simulink model "PubIfDecisionLM_MDL"  (R2020b)
settings: configuration reference "DspaceConfig" (kept outside this file)
PostLoadFcn:
  | if any(exist('dsrtsu_mdlpostloadfcn', 'file') ~= 0), dsrtsu_mdlpostloadfcn('Execute', bdroot); end
InitFcn:
  | , if any(exist('dsmpb_private', 'file') ~= 0), dsmpb_private('dsmpb_mdlclblib', 'Init', bdroot); end,
undefined symbols (not defined in the file or in its folder): OFM_OBJ_FUSIONTYPE_E, OFM_OBJ_MOVINGSTATE_E, OFM_OBJ_ORIENTATION_E, OFM_OBJ_TYPE_E, P_LM_Cyc, P_LM_EMLHistKapRcdBufSize, P_LM_EMLHistTrajBaseDis, P_LM_EMLHistTrajPNum, P_LM_EMLKapCorrMaxThre, P_LM_EMLMinKapThre, P_LM_EMLPathDisDiffThre, P_LM_EMLQuaFiltPar, P_LM_EMLTurnActKapThre, P_LM_EMLValidQuaThre, P_LM_FntPath1Disgap, P_LM_FntPath1MinDis, P_LM_FntPath1Timegap, P_LM_FntPath2Disgap, P_LM_FntPath2MinDis, P_LM_FntPath2Timegap, P_LM_FntPath3Disgap, P_LM_FntPath3MinDis, P_LM_FntPath3Timegap, P_LM_FusBLParFiltP, P_LM_FusEVDifC2Thre, P_LM_FusEVOPath1AllVSLDisThre, P_LM_FusEVOPath1AllVSLLostNumThre, P_LM_FusEVOPath1AllVSLQuaThre, P_LM_FusEVOPath1OTLFacNLC, P_LM_FusOTLQuaThre, P_LM_FusOTLSW, P_LM_FusParC0Index, P_LM_FusParC1Index, P_LM_FusParC2Index, P_LM_FusParC3Index, P_LM_FusVSLQuaThre, P_LM_FusVSLSW, P_LM_FusVSLValidSteerWheerAngThre, P_LM_FusVSLValidVxvThre, P_LM_LaneWidth, P_LM_OTLBufTPInfoEvaFactor, P_LM_OTLObjNum, P_LM_OTLObjSelectAgeThre, P_LM_OTLObjSelectDxAssessVx, P_LM_OTLObjSelectDxThre, P_LM_OTLObjSelectVxThre, P_LM_OTLObjSelectVyAssessDx, P_LM_OTLObjSelectVyThre, P_LM_OTLTrajPntBaseDis, P_LM_OTLTrajStdThre, P_LM_VSLAvailLineNum, P_LM_VSLBLSDiffThre, P_LM_VSLBLSDisRatio, P_LM_VSLFusBLParFiltP_C1, P_LM_VSLFusBLParFiltP_C2, P_LM_VSLFusBLParFiltP_C3, P_LM_VSLFusBLParFiltP_Quality, P_LM_VSLHistTrajBaseDis, P_LM_VSLHistTrajPNum, P_LM_VSLLCC0diff ... (+18)
libraries: simulink x145, LM_LIB x43
(part 15 of 24)

== system PubIfDecisionLM_MDL/Subsystem2/LM_Fusion1/LM_Fus_BLConnectivityCheck/LM_Fus_BLFntPahtConnectivityCheck/LM_Fus_BLFntPahtConnectivityCheck/LM_Fus_BLFntPath2Info/LM_Fus_BLFntPath2C0Adju ==
  LM_FusBLFntPath1C0 : Inport
  LM_FusBLFntPath1C1 : Inport  Port=2
  LM_FusBLFntPath1C2 : Inport  Port=3
  LM_FusBLFntPath1C3 : Inport  Port=4
  LM_FntPath1Dis : Inport  Port=5
  LM_FusBLFntPath2C0BefAduj : Inport  Port=6
  LM_FusBLFntPath2C1 : Inport  Port=7
  LM_FusBLFntPath2C2 : Inport  Port=8
  LM_FusBLFntPath2C3 : Inport  Port=9
  LM_Fus_BLFntPaht1EndPosCalc : Subsystem
  LM_Fus_BLFntPath2C0Adju : Subsystem
  LM_Fus_BLFntPath2StartPosCalc : Subsystem
  LM_FusBLFntPath2C0Aduj : Outport
  wires:
  LM_FusBLFntPath1C0/1 -> LM_Fus_BLFntPaht1EndPosCalc/1(LM_FusBLFntPath1C0)
  LM_FusBLFntPath1C1/1 -> LM_Fus_BLFntPaht1EndPosCalc/2(LM_FusBLFntPath1C1)
  LM_FusBLFntPath1C2/1 -> LM_Fus_BLFntPaht1EndPosCalc/3(LM_FusBLFntPath1C2)
  LM_FusBLFntPath1C3/1 -> LM_Fus_BLFntPaht1EndPosCalc/4(LM_FusBLFntPath1C3)
  LM_FntPath1Dis/1 -> LM_Fus_BLFntPath2StartPosCalc/1(LM_FntPath1Dis), LM_Fus_BLFntPaht1EndPosCalc/5(LM_FntPath1Dis)
  LM_FusBLFntPath2C1/1 -> LM_Fus_BLFntPath2StartPosCalc/2(LM_FusBLFntPath2C1)
  LM_FusBLFntPath2C2/1 -> LM_Fus_BLFntPath2StartPosCalc/3(LM_FusBLFntPath2C2)
  LM_FusBLFntPath2C3/1 -> LM_Fus_BLFntPath2StartPosCalc/4(LM_FusBLFntPath2C3)
  LM_FusBLFntPath2C0BefAduj/1 -> LM_Fus_BLFntPath2C0Adju/3(LM_FusBLFntPath2C0BefAduj), LM_Fus_BLFntPath2StartPosCalc/5(LM_FusBLFntPath2C0BefAduj)
  LM_Fus_BLFntPaht1EndPosCalc/1(LM_FusBLFntPaht1EndPosdy) -> LM_Fus_BLFntPath2C0Adju/1(LM_FusBLFntPaht1EndPosdy)
  LM_Fus_BLFntPath2StartPosCalc/1(LM_FusBLFntPaht2StartPosdy) -> LM_Fus_BLFntPath2C0Adju/2(LM_FusBLFntPaht2StartPosdy)
  LM_Fus_BLFntPath2C0Adju/1(LM_FusBLFntPath2C0Aduj) -> LM_FusBLFntPath2C0Aduj/1

== system PubIfDecisionLM_MDL/Subsystem2/LM_Fusion1/LM_Fus_BLConnectivityCheck/LM_Fus_BLFntPahtConnectivityCheck/LM_Fus_BLFntPahtConnectivityCheck/LM_Fus_BLFntPath2Info/LM_Fus_BLFntPath2Info ==
  LM_FusBLFntPath2C0Aduj : Inport
  LM_FusBLFntPath2C1 : Inport  Port=2
  LM_FusBLFntPath2C2 : Inport  Port=3
  LM_FusBLFntPath2C3 : Inport  Port=4
  LM_FusBLFntPath2Quality : Inport  Port=5
  Signal Conversion{,1..4} (5 alike) : SignalConversion  OverrideOpt=off
  LM_FusBLFntPath2C0Adju : Outport
  LM_FusBLFntPath2C1Adju : Outport  Port=2
  LM_FusBLFntPath2C2Adju : Outport  Port=3
  LM_FusBLFntPath2C3Adju : Outport  Port=4
  LM_FusBLFntPath2QualityAdju : Outport  Port=5
  wires:
  LM_FusBLFntPath2Quality/1 -> Signal Conversion4/1
  LM_FusBLFntPath2C2/1 -> Signal Conversion2/1
  LM_FusBLFntPath2C1/1 -> Signal Conversion1/1
  LM_FusBLFntPath2C0Aduj/1 -> Signal Conversion/1
  LM_FusBLFntPath2C3/1 -> Signal Conversion3/1
  Signal Conversion/1 -> LM_FusBLFntPath2C0Adju/1  "LM_FusBLFntPath2C0Adju"
  Signal Conversion2/1 -> LM_FusBLFntPath2C2Adju/1  "LM_FusBLFntPath2C2Adju"
  Signal Conversion4/1 -> LM_FusBLFntPath2QualityAdju/1  "LM_FusBLFntPath2QualityAdju"
  Signal Conversion3/1 -> LM_FusBLFntPath2C3Adju/1  "LM_FusBLFntPath2C3Adju"
  Signal Conversion1/1 -> LM_FusBLFntPath2C1Adju/1  "LM_FusBLFntPath2C1Adju"

== system PubIfDecisionLM_MDL/Subsystem2/LM_Fusion1/LM_Fus_BLConnectivityCheck/LM_Fus_BLFntPahtConnectivityCheck/LM_Fus_BLFntPahtConnectivityCheck/LM_Fus_BLFntPath3Info/LM_Fus_BLFntPath2C0Adju ==
  LM_FusBLFntPath2C0 : Inport
  LM_FusBLFntPath2C1 : Inport  Port=2
  LM_FusBLFntPath2C2 : Inport  Port=3
  LM_FusBLFntPath2C3 : Inport  Port=4
  LM_FntPath2Dis : Inport  Port=5
  LM_FusBLFntPath3C0BefAduj : Inport  Port=6
  LM_FusBLFntPath3C1 : Inport  Port=7
  LM_FusBLFntPath3C2 : Inport  Port=8
  LM_FusBLFntPath3C3 : Inport  Port=9
  LM_Fus_BLFntPaht2EndPosCalc : Subsystem
  LM_Fus_BLFntPath3C0Adju : Subsystem
  LM_Fus_BLFntPath3StartPosCalc : Subsystem
  LM_FusBLFntPath3C0Aduj : Outport
  wires:
  LM_FusBLFntPath2C0/1 -> LM_Fus_BLFntPaht2EndPosCalc/1(LM_FusBLFntPath2C0)
  LM_FusBLFntPath2C1/1 -> LM_Fus_BLFntPaht2EndPosCalc/2(LM_FusBLFntPath2C1)
  LM_FusBLFntPath2C2/1 -> LM_Fus_BLFntPaht2EndPosCalc/3(LM_FusBLFntPath2C2)
  LM_FusBLFntPath2C3/1 -> LM_Fus_BLFntPaht2EndPosCalc/4(LM_FusBLFntPath2C3)
  LM_FntPath2Dis/1 -> LM_Fus_BLFntPath3StartPosCalc/1(LM_FntPath2Dis), LM_Fus_BLFntPaht2EndPosCalc/5(LM_FntPath2Dis)
  LM_FusBLFntPath3C1/1 -> LM_Fus_BLFntPath3StartPosCalc/2(LM_FusBLFntPath3C1)
  LM_FusBLFntPath3C2/1 -> LM_Fus_BLFntPath3StartPosCalc/3(LM_FusBLFntPath3C2)
  LM_FusBLFntPath3C3/1 -> LM_Fus_BLFntPath3StartPosCalc/4(LM_FusBLFntPath3C3)
  LM_FusBLFntPath3C0BefAduj/1 -> LM_Fus_BLFntPath3C0Adju/3(LM_FusBLFntPath3C0BefAduj), LM_Fus_BLFntPath3StartPosCalc/5(LM_FusBLFntPath3C0BefAduj)
  LM_Fus_BLFntPaht2EndPosCalc/1(LM_FusBLFntPaht2EndPosdy) -> LM_Fus_BLFntPath3C0Adju/1(LM_FusBLFntPaht2EndPosdy)
  LM_Fus_BLFntPath3StartPosCalc/1(LM_FusBLFntPaht3StartPosdy) -> LM_Fus_BLFntPath3C0Adju/2(LM_FusBLFntPaht3StartPosdy)
  LM_Fus_BLFntPath3C0Adju/1(LM_FusBLFntPath3C0Aduj) -> LM_FusBLFntPath3C0Aduj/1

== system PubIfDecisionLM_MDL/Subsystem2/LM_Fusion1/LM_Fus_BLConnectivityCheck/LM_Fus_BLFntPahtConnectivityCheck/LM_Fus_BLFntPahtConnectivityCheck/LM_Fus_BLFntPath3Info/LM_Fus_BLFntPath2Info ==
  LM_FusBLFntPath3C0Aduj : Inport
  LM_FusBLFntPath3C1 : Inport  Port=2
  LM_FusBLFntPath3C2 : Inport  Port=3
  LM_FusBLFntPath3C3 : Inport  Port=4
  LM_FusBLFntPath3Quality : Inport  Port=5
  Signal Conversion{,1..4} (5 alike) : SignalConversion  OverrideOpt=off
  LM_FusBLFntPath3C0Adju : Outport
  LM_FusBLFntPath3C1Adju : Outport  Port=2
  LM_FusBLFntPath3C2Adju : Outport  Port=3
  LM_FusBLFntPath3C3Adju : Outport  Port=4
  LM_FusBLFntPath3QualityAdju : Outport  Port=5
  wires:
  Signal Conversion4/1 -> LM_FusBLFntPath3QualityAdju/1  "LM_FusBLFntPath3QualityAdju"
  Signal Conversion2/1 -> LM_FusBLFntPath3C2Adju/1  "LM_FusBLFntPath3C2Adju"
  Signal Conversion/1 -> LM_FusBLFntPath3C0Adju/1  "LM_FusBLFntPath3C0Adju"
  Signal Conversion3/1 -> LM_FusBLFntPath3C3Adju/1  "LM_FusBLFntPath3C3Adju"
  Signal Conversion1/1 -> LM_FusBLFntPath3C1Adju/1  "LM_FusBLFntPath3C1Adju"
  LM_FusBLFntPath3C0Aduj/1 -> Signal Conversion/1
  LM_FusBLFntPath3C1/1 -> Signal Conversion1/1
  LM_FusBLFntPath3C2/1 -> Signal Conversion2/1
  LM_FusBLFntPath3C3/1 -> Signal Conversion3/1
  LM_FusBLFntPath3Quality/1 -> Signal Conversion4/1

== system PubIfDecisionLM_MDL/Subsystem2/LM_Fusion1/LM_Fus_BLConnectivityCheck/LM_Fus_BLRearPahtConnectivityCheck/LM_Fus_BLRearPahtConnectivityCheck/LM_Fus_BLFntPath2Info/LM_Fus_BLFntPath2C0Adju ==
  LM_FusBLFntPath1C0 : Inport
  LM_FusBLFntPath1C1 : Inport  Port=2
  LM_FusBLFntPath1C2 : Inport  Port=3
  LM_FusBLFntPath1C3 : Inport  Port=4
  LM_FntPath1Dis : Inport  Port=5
  LM_FusBLFntPath2C0BefAduj : Inport  Port=6
  LM_FusBLFntPath2C1 : Inport  Port=7
  LM_FusBLFntPath2C2 : Inport  Port=8
  LM_FusBLFntPath2C3 : Inport  Port=9
  LM_Fus_BLFntPaht1EndPosCalc : Subsystem
  LM_Fus_BLFntPath2C0Adju : Subsystem
  LM_Fus_BLFntPath2StartPosCalc : Subsystem
  LM_FusBLFntPath2C0Aduj : Outport
  wires:
  LM_FusBLFntPath1C0/1 -> LM_Fus_BLFntPaht1EndPosCalc/1(LM_FusBLFntPath1C0)
  LM_FusBLFntPath1C1/1 -> LM_Fus_BLFntPaht1EndPosCalc/2(LM_FusBLFntPath1C1)
  LM_FusBLFntPath1C2/1 -> LM_Fus_BLFntPaht1EndPosCalc/3(LM_FusBLFntPath1C2)
  LM_FusBLFntPath1C3/1 -> LM_Fus_BLFntPaht1EndPosCalc/4(LM_FusBLFntPath1C3)
  LM_FntPath1Dis/1 -> LM_Fus_BLFntPath2StartPosCalc/1(LM_FntPath1Dis), LM_Fus_BLFntPaht1EndPosCalc/5(LM_FntPath1Dis)
  LM_FusBLFntPath2C1/1 -> LM_Fus_BLFntPath2StartPosCalc/2(LM_FusBLFntPath2C1)
  LM_FusBLFntPath2C2/1 -> LM_Fus_BLFntPath2StartPosCalc/3(LM_FusBLFntPath2C2)
  LM_FusBLFntPath2C3/1 -> LM_Fus_BLFntPath2StartPosCalc/4(LM_FusBLFntPath2C3)
  LM_FusBLFntPath2C0BefAduj/1 -> LM_Fus_BLFntPath2C0Adju/3(LM_FusBLFntPath2C0BefAduj), LM_Fus_BLFntPath2StartPosCalc/5(LM_FusBLFntPath2C0BefAduj)
  LM_Fus_BLFntPaht1EndPosCalc/1(LM_FusBLFntPaht1EndPosdy) -> LM_Fus_BLFntPath2C0Adju/1(LM_FusBLFntPaht1EndPosdy)
  LM_Fus_BLFntPath2StartPosCalc/1(LM_FusBLFntPaht2StartPosdy) -> LM_Fus_BLFntPath2C0Adju/2(LM_FusBLFntPaht2StartPosdy)
  LM_Fus_BLFntPath2C0Adju/1(LM_FusBLFntPath2C0Aduj) -> LM_FusBLFntPath2C0Aduj/1

== system PubIfDecisionLM_MDL/Subsystem2/LM_Fusion1/LM_Fus_BLConnectivityCheck/LM_Fus_BLRearPahtConnectivityCheck/LM_Fus_BLRearPahtConnectivityCheck/LM_Fus_BLFntPath2Info/LM_Fus_BLFntPath2Info ==
  LM_FusBLFntPath2C0Aduj : Inport
  LM_FusBLFntPath2C1 : Inport  Port=2
  LM_FusBLFntPath2C2 : Inport  Port=3
  LM_FusBLFntPath2C3 : Inport  Port=4
  LM_FusBLFntPath2Quality : Inport  Port=5
  Signal Conversion{,1..4} (5 alike) : SignalConversion  OverrideOpt=off
  LM_FusBLRearPath2C0Adju : Outport
  LM_FusBLRearPath2C1Adju : Outport  Port=2
  LM_FusBLRearPath2C2Adju : Outport  Port=3
  LM_FusBLRearPath2C3Adju : Outport  Port=4
  LM_FusBLRearPath2QualityAdju : Outport  Port=5
  wires:
  LM_FusBLFntPath2C2/1 -> Signal Conversion2/1
  Signal Conversion3/1 -> LM_FusBLRearPath2C3Adju/1  "LM_FusBLRearPath2C3Adju"
  LM_FusBLFntPath2C0Aduj/1 -> Signal Conversion/1
  Signal Conversion4/1 -> LM_FusBLRearPath2QualityAdju/1  "LM_FusBLRearPath2QualityAdju"
  Signal Conversion/1 -> LM_FusBLRearPath2C0Adju/1  "LM_FusBLRearPath2C0Adju"
  Signal Conversion2/1 -> LM_FusBLRearPath2C2Adju/1  "LM_FusBLRearPath2C2Adju"
  LM_FusBLFntPath2C3/1 -> Signal Conversion3/1
  LM_FusBLFntPath2C1/1 -> Signal Conversion1/1
  Signal Conversion1/1 -> LM_FusBLRearPath2C1Adju/1  "LM_FusBLRearPath2C1Adju"
  LM_FusBLFntPath2Quality/1 -> Signal Conversion4/1

== system PubIfDecisionLM_MDL/Subsystem2/LM_Fusion1/LM_Fus_BLConnectivityCheck/LM_Fus_BLRearPahtConnectivityCheck/LM_Fus_BLRearPahtConnectivityCheck/LM_Fus_BLFntPath3Info/LM_Fus_BLFntPath2Info ==
  LM_FusBLFntPath3C0Check : Inport
  LM_FusBLFntPath3C1 : Inport  Port=2
  LM_FusBLFntPath3C2 : Inport  Port=3
  LM_FusBLFntPath3C3 : Inport  Port=4
  LM_FusBLFntPath3Quality : Inport  Port=5
  Signal Conversion{,1..4} (5 alike) : SignalConversion  OverrideOpt=off
  LM_FusBLRearPath3C0Adju : Outport
  LM_FusBLRearPath3C1Adju : Outport  Port=2
  LM_FusBLRearPath3C2Adju : Outport  Port=3
  LM_FusBLRearPath3C3Adju : Outport  Port=4
  LM_FusBLRearPath3QualityAdju : Outport  Port=5
  wires:
  LM_FusBLFntPath3C0Check/1 -> Signal Conversion/1
  Signal Conversion1/1 -> LM_FusBLRearPath3C1Adju/1  "LM_FusBLRearPath3C1Adju"
  Signal Conversion3/1 -> LM_FusBLRearPath3C3Adju/1  "LM_FusBLRearPath3C3Adju"
  LM_FusBLFntPath3Quality/1 -> Signal Conversion4/1
  Signal Conversion4/1 -> LM_FusBLRearPath3QualityAdju/1  "LM_FusBLRearPath3QualityAdju"
  LM_FusBLFntPath3C3/1 -> Signal Conversion3/1
  LM_FusBLFntPath3C2/1 -> Signal Conversion2/1
  Signal Conversion2/1 -> LM_FusBLRearPath3C2Adju/1  "LM_FusBLRearPath3C2Adju"
  LM_FusBLFntPath3C1/1 -> Signal Conversion1/1
  Signal Conversion/1 -> LM_FusBLRearPath3C0Adju/1  "LM_FusBLRearPath3C0Adju"

== system PubIfDecisionLM_MDL/Subsystem2/LM_Fusion1/LM_Fus_BLConnectivityCheck/LM_Fus_BLRearPahtConnectivityCheck/LM_Fus_BLRearPahtConnectivityCheck/LM_Fus_BLFntPath3Info/LM_Fus_BLRearPath3C0Adju ==
  LM_FusBLFntPath2C0 : Inport
  LM_FusBLFntPath2C1 : Inport  Port=2
  LM_FusBLFntPath2C2 : Inport  Port=3
  LM_FusBLFntPath2C3 : Inport  Port=4
  LM_FntPath2Dis : Inport  Port=5
  LM_FusBLFntPath3C0BefAduj : Inport  Port=6
  LM_FusBLFntPath3C1 : Inport  Port=7
  LM_FusBLFntPath3C2 : Inport  Port=8
  LM_FusBLFntPath3C3 : Inport  Port=9
  LM_Fus_BLFntPaht2EndPosCalc : Subsystem
  LM_Fus_BLFntPath3C0Adju : Subsystem
  LM_Fus_BLFntPath3StartPosCalc : Subsystem
  LM_FusBLFntPath3C0Check : Outport
  wires:
  LM_FusBLFntPath2C0/1 -> LM_Fus_BLFntPaht2EndPosCalc/1(LM_FusBLFntPath2C0)
  LM_FusBLFntPath2C1/1 -> LM_Fus_BLFntPaht2EndPosCalc/2(LM_FusBLFntPath2C1)
  LM_FusBLFntPath2C2/1 -> LM_Fus_BLFntPaht2EndPosCalc/3(LM_FusBLFntPath2C2)
  LM_FusBLFntPath2C3/1 -> LM_Fus_BLFntPaht2EndPosCalc/4(LM_FusBLFntPath2C3)
  LM_FntPath2Dis/1 -> LM_Fus_BLFntPath3StartPosCalc/1(LM_FntPath2Dis), LM_Fus_BLFntPaht2EndPosCalc/5(LM_FntPath2Dis)
  LM_FusBLFntPath3C1/1 -> LM_Fus_BLFntPath3StartPosCalc/2(LM_FusBLFntPath3C1)
  LM_FusBLFntPath3C2/1 -> LM_Fus_BLFntPath3StartPosCalc/3(LM_FusBLFntPath3C2)
  LM_FusBLFntPath3C3/1 -> LM_Fus_BLFntPath3StartPosCalc/4(LM_FusBLFntPath3C3)
  LM_FusBLFntPath3C0BefAduj/1 -> LM_Fus_BLFntPath3C0Adju/3(LM_FusBLFntPath3C0BefAduj), LM_Fus_BLFntPath3StartPosCalc/5(LM_FusBLFntPath3C0BefAduj)
  LM_Fus_BLFntPaht2EndPosCalc/1(LM_FusBLFntPaht2EndPosdy) -> LM_Fus_BLFntPath3C0Adju/1(LM_FusBLFntPaht2EndPosdy)
  LM_Fus_BLFntPath3StartPosCalc/1(LM_FusBLFntPaht3StartPosdy) -> LM_Fus_BLFntPath3C0Adju/2(LM_FusBLFntPaht3StartPosdy)
  LM_Fus_BLFntPath3C0Adju/1(LM_FusBLFntPath3C0Check) -> LM_FusBLFntPath3C0Check/1

== system PubIfDecisionLM_MDL/Subsystem2/LM_OTL/LM_OTL_MovObjTrajRecord3/LM_OTL_BufTPCC/Subsystem/LM_OTLHostBufCoordinateConvert/If Action Subsystem ==
  LM_OTLOffsetX : Inport
  LM_OTLOffsetY : Inport  Port=2
  LM_OTLOffsetAng : Inport  Port=3
  LM_OTLBufE1DxVectK1 : Inport  Port=4
  LM_OTLBufE1DyVectK1 : Inport  Port=5
  LM_OTLBufE2DxVectK1 : Inport  Port=6
  LM_OTLBufE2DyVectK1 : Inport  Port=7
  Action Port : ActionPort  ActionPortLabel=if(u1 == 0)
  For Each Subsystem : Subsystem  TreatAsAtomicUnit=on
  LM_OTLBufE1DxVectK1Adju : Outport
  LM_OTLBufE1DyVectK1Adju : Outport  Port=2
  LM_OTLBufE2DxVectK1Adju : Outport  Port=3
  LM_OTLBufE2DyVectK1Adju : Outport  Port=4
  wires:
  For Each Subsystem/3(LM_OTLBufE2DxVectK1Adju) -> LM_OTLBufE2DxVectK1Adju/1
  For Each Subsystem/4(LM_OTLBufE2DyVectK1Adju) -> LM_OTLBufE2DyVectK1Adju/1
  For Each Subsystem/1(LM_OTLBufE1DxVectK1Adju) -> LM_OTLBufE1DxVectK1Adju/1
  For Each Subsystem/2(LM_OTLBufE1DyVectK1Adju) -> LM_OTLBufE1DyVectK1Adju/1
  LM_OTLBufE2DyVectK1/1 -> For Each Subsystem/7(LM_OTLBufE2DyVectK1)
  LM_OTLBufE2DxVectK1/1 -> For Each Subsystem/6(LM_OTLBufE2DxVectK1)
  LM_OTLBufE1DxVectK1/1 -> For Each Subsystem/4(LM_OTLBufE1DxVectK1)
  LM_OTLBufE1DyVectK1/1 -> For Each Subsystem/5(LM_OTLBufE1DyVectK1)
  LM_OTLOffsetAng/1 -> For Each Subsystem/3(LM_OTLOffsetAng)
  LM_OTLOffsetY/1 -> For Each Subsystem/2(LM_OTLOffsetY)
  LM_OTLOffsetX/1 -> For Each Subsystem/1(LM_OTLOffsetX)

== system PubIfDecisionLM_MDL/Subsystem2/LM_OTL/LM_OTL_MovObjTrajRecord3/LM_OTL_BufTPCC/Subsystem/LM_OTLHostBufCoordinateConvert/If Action Subsystem1 ==
  LM_OTLBufE1DxVectK1 : Inport
  LM_OTLBufE1DyVectK1 : Inport  Port=2
  LM_OTLBufE2DxVectK1 : Inport  Port=3
  LM_OTLBufE2DyVectK1 : Inport  Port=4
  Action Port : ActionPort  ActionPortLabel=else
  LM_OTLBufE1DxVectK1Adju : Outport
  LM_OTLBufE1DyVectK1Adju : Outport  Port=2
  LM_OTLBufE2DxVectK1Adju : Outport  Port=3
  LM_OTLBufE2DyVectK1Adju : Outport  Port=4
  wires:
  LM_OTLBufE1DxVectK1/1 -> LM_OTLBufE1DxVectK1Adju/1
  LM_OTLBufE1DyVectK1/1 -> LM_OTLBufE1DyVectK1Adju/1
  LM_OTLBufE2DxVectK1/1 -> LM_OTLBufE2DxVectK1Adju/1
  LM_OTLBufE2DyVectK1/1 -> LM_OTLBufE2DyVectK1Adju/1

== system PubIfDecisionLM_MDL/Subsystem2/LM_OTL/LM_OTL_MovObjTrajRecord3/LM_OTL_BufTPCC/Subsystem/LM_OTLLeBufCoordinateConvert/If Action Subsystem ==
  LM_OTLOffsetX : Inport
  LM_OTLOffsetY : Inport  Port=2
  LM_OTLOffsetAng : Inport  Port=3
  LM_OTLBufL1DxVectK1 : Inport  Port=4
  LM_OTLBufL1DyVectK1 : Inport  Port=5
  LM_OTLBufL2DxVectK1 : Inport  Port=6
  LM_OTLBufL2DyVectK1 : Inport  Port=7
  Action Port : ActionPort  ActionPortLabel=if(u1 == 0)
  For Each Subsystem : Subsystem  TreatAsAtomicUnit=on
  LM_OTLBufL1DxVectK1Adju : Outport
  LM_OTLBufL1DyVectK1Adju : Outport  Port=2
  LM_OTLBufL2DxVectK1Adju : Outport  Port=3
  LM_OTLBufL2DyVectK1Adju : Outport  Port=4
  wires:
  For Each Subsystem/3(LM_OTLBufL2DxVectK1Adju) -> LM_OTLBufL2DxVectK1Adju/1
  For Each Subsystem/4(LM_OTLBufL2DyVectK1Adju) -> LM_OTLBufL2DyVectK1Adju/1
  For Each Subsystem/1(LM_OTLBufL1DxVectK1Adju) -> LM_OTLBufL1DxVectK1Adju/1
  For Each Subsystem/2(LM_OTLBufL1DyVectK1Adju) -> LM_OTLBufL1DyVectK1Adju/1
  LM_OTLBufL2DyVectK1/1 -> For Each Subsystem/7(LM_OTLBufL2DyVectK1)
  LM_OTLBufL2DxVectK1/1 -> For Each Subsystem/6(LM_OTLBufL2DxVectK1)
  LM_OTLBufL1DxVectK1/1 -> For Each Subsystem/4(LM_OTLBufL1DxVectK1)
  LM_OTLBufL1DyVectK1/1 -> For Each Subsystem/5(LM_OTLBufL1DyVectK1)
  LM_OTLOffsetAng/1 -> For Each Subsystem/3(LM_OTLOffsetAng)
  LM_OTLOffsetY/1 -> For Each Subsystem/2(LM_OTLOffsetY)
  LM_OTLOffsetX/1 -> For Each Subsystem/1(LM_OTLOffsetX)

== system PubIfDecisionLM_MDL/Subsystem2/LM_OTL/LM_OTL_MovObjTrajRecord3/LM_OTL_BufTPCC/Subsystem/LM_OTLLeBufCoordinateConvert/If Action Subsystem1 ==
  LM_OTLBufL1DxVectK1 : Inport
  LM_OTLBufL1DyVectK1 : Inport  Port=2
  LM_OTLBufL2DxVectK1 : Inport  Port=3
  LM_OTLBufL2DyVectK1 : Inport  Port=4
  Action Port : ActionPort  ActionPortLabel=else
  LM_OTLBufL1DxVectK1Adju : Outport
  LM_OTLBufL1DyVectK1Adju : Outport  Port=2
  LM_OTLBufL2DxVectK1Adju : Outport  Port=3
  LM_OTLBufL2DyVectK1Adju : Outport  Port=4
  wires:
  LM_OTLBufL1DxVectK1/1 -> LM_OTLBufL1DxVectK1Adju/1
  LM_OTLBufL1DyVectK1/1 -> LM_OTLBufL1DyVectK1Adju/1
  LM_OTLBufL2DxVectK1/1 -> LM_OTLBufL2DxVectK1Adju/1
  LM_OTLBufL2DyVectK1/1 -> LM_OTLBufL2DyVectK1Adju/1

== system PubIfDecisionLM_MDL/Subsystem2/LM_OTL/LM_OTL_MovObjTrajRecord3/LM_OTL_BufTPCC/Subsystem/LM_OTLRiBufCoordinateConvert/If Action Subsystem ==
  LM_OTLOffsetX : Inport
  LM_OTLOffsetY : Inport  Port=2
  LM_OTLOffsetAng : Inport  Port=3
  LM_OTLBufR1DxVectK1 : Inport  Port=4
  LM_OTLBufR1DyVectK1 : Inport  Port=5
  LM_OTLBufR2DxVectK1 : Inport  Port=6
  LM_OTLBufR2DyVectK1 : Inport  Port=7
  Action Port : ActionPort  ActionPortLabel=if(u1 == 0)
  For Each Subsystem : Subsystem  TreatAsAtomicUnit=on
  LM_OTLBufR1DxVectK1Adju : Outport
  LM_OTLBufR1DyVectK1Adju : Outport  Port=2
  LM_OTLBufR2DxVectK1Adju : Outport  Port=3
  LM_OTLBufR2DyVectK1Adju : Outport  Port=4
  wires:
  For Each Subsystem/3(LM_OTLBufR2DxVectK1Adju) -> LM_OTLBufR2DxVectK1Adju/1
  For Each Subsystem/4(LM_OTLBufR2DyVectK1Adju) -> LM_OTLBufR2DyVectK1Adju/1
  For Each Subsystem/1(LM_OTLBufR1DxVectK1Adju) -> LM_OTLBufR1DxVectK1Adju/1
  For Each Subsystem/2(LM_OTLBufR1DyVectK1Adju) -> LM_OTLBufR1DyVectK1Adju/1
  LM_OTLBufR2DyVectK1/1 -> For Each Subsystem/7(LM_OTLBufR2DyVectK1)
  LM_OTLBufR2DxVectK1/1 -> For Each Subsystem/6(LM_OTLBufR2DxVectK1)
  LM_OTLBufR1DxVectK1/1 -> For Each Subsystem/4(LM_OTLBufR1DxVectK1)
  LM_OTLBufR1DyVectK1/1 -> For Each Subsystem/5(LM_OTLBufR1DyVectK1)
  LM_OTLOffsetAng/1 -> For Each Subsystem/3(LM_OTLOffsetAng)
  LM_OTLOffsetY/1 -> For Each Subsystem/2(LM_OTLOffsetY)
  LM_OTLOffsetX/1 -> For Each Subsystem/1(LM_OTLOffsetX)

== system PubIfDecisionLM_MDL/Subsystem2/LM_OTL/LM_OTL_MovObjTrajRecord3/LM_OTL_BufTPCC/Subsystem/LM_OTLRiBufCoordinateConvert/If Action Subsystem1 ==
  LM_OTLBufR1DxVectK1 : Inport
  LM_OTLBufR1DyVectK1 : Inport  Port=2
  LM_OTLBufR2DxVectK1 : Inport  Port=3
  LM_OTLBufR2DyVectK1 : Inport  Port=4
  Action Port : ActionPort  ActionPortLabel=else
  LM_OTLBufR1DxVectK1Adju : Outport
  LM_OTLBufR1DyVectK1Adju : Outport  Port=2
  LM_OTLBufR2DxVectK1Adju : Outport  Port=3
  LM_OTLBufR2DyVectK1Adju : Outport  Port=4
  wires:
  LM_OTLBufR1DxVectK1/1 -> LM_OTLBufR1DxVectK1Adju/1
  LM_OTLBufR1DyVectK1/1 -> LM_OTLBufR1DyVectK1Adju/1
  LM_OTLBufR2DxVectK1/1 -> LM_OTLBufR2DxVectK1Adju/1
  LM_OTLBufR2DyVectK1/1 -> LM_OTLBufR2DyVectK1Adju/1

== system PubIfDecisionLM_MDL/Subsystem2/LM_OTL/LM_OTL_MovObjTrajRecord3/LM_OTL_MovObjSelc/LM_OTL_MovObjInterestedSelc/LM_OTL_ObjSelcIndexCalc/LM_OTL_ObjSelcCalc ==
  LeObjSelcDxInfo : Inport
  HostObjSlecDxInfo : Inport  Port=2
  RigObjSlecDxInfo : Inport  Port=3
  C_LM_ObjNum : Inport  Port=4
  LM_OTL_HostObjSelc : Subsystem
  LM_OTL_LeObjSelc : Subsystem
  LM_OTL_RigObjSelc : Subsystem
  LeObj1CheckInfo : Outport
  LeObj2CheckInfo : Outport  Port=2
  HostObj1CheckInfo : Outport  Port=3
  HostObj2CheckInfo : Outport  Port=4
  RigObj1CheckInfo : Outport  Port=5
  RigObj2CheckInfo : Outport  Port=6
  wires:
  HostObjSlecDxInfo/1 -> LM_OTL_HostObjSelc/2(HostObjSelcDxInfo)
  RigObjSlecDxInfo/1 -> LM_OTL_RigObjSelc/2(RigObjSelcDxInfo)
  LM_OTL_LeObjSelc/2(LeObj2Index) -> LeObj2CheckInfo/1
  LeObjSelcDxInfo/1 -> LM_OTL_LeObjSelc/2(LeObjSelcDxInfo)
  LM_OTL_RigObjSelc/1(RigObj1Index) -> RigObj1CheckInfo/1
  LM_OTL_HostObjSelc/2(HostObj2Index) -> HostObj2CheckInfo/1
  LM_OTL_RigObjSelc/2(RigObj2Index) -> RigObj2CheckInfo/1
  C_LM_ObjNum/1 -> LM_OTL_HostObjSelc/1(C_LM_ObjNum), LM_OTL_RigObjSelc/1(C_LM_ObjNum), LM_OTL_LeObjSelc/1(C_LM_ObjNum)
  LM_OTL_HostObjSelc/1(HostObj1Index) -> HostObj1CheckInfo/1
  LM_OTL_LeObjSelc/1(LeObj1Index) -> LeObj1CheckInfo/1

== system PubIfDecisionLM_MDL/Subsystem2/LM_OTL/LM_OTL_MovObjTrajRecord3/LM_OTL_MovObjSelc/LM_OTL_MovObjInterestedSelc/LM_OTL_ObjSelcIndexCalc/LM_OTL_ObjSelcInfoOpt ==
  ObjSelcDxInfo : Inport
  ObjSelcDyInfo : Inport  Port=2
  HostObjSelcInfoOpt : Subsystem
  LeObjSelcInfoOpt : Subsystem
  RigObjSelcInfoOpt : Subsystem
  LeObjSelcDxInfo : Outport
  HostObjSlecDxInfo : Outport  Port=2
  RigObjSlecDxInfo : Outport  Port=3
  wires:
  RigObjSelcInfoOpt/1(RigObjSlecDxInfo) -> RigObjSlecDxInfo/1
  HostObjSelcInfoOpt/1(HostObjSlecDxInfo) -> HostObjSlecDxInfo/1
  LeObjSelcInfoOpt/1(LeObjSelcDxInfo) -> LeObjSelcDxInfo/1
  ObjSelcDyInfo/1 -> HostObjSelcInfoOpt/2(ObjSelcDyInfo), RigObjSelcInfoOpt/2(ObjSelcDyInfo), LeObjSelcInfoOpt/2(ObjSelcDyInfo)
  ObjSelcDxInfo/1 -> HostObjSelcInfoOpt/1(ObjSelcDxInfo), RigObjSelcInfoOpt/1(ObjSelcDxInfo), LeObjSelcInfoOpt/1(ObjSelcDxInfo)

== system PubIfDecisionLM_MDL/Subsystem2/LM_OTL/LM_OTL_MovObjTrajRecord3/LM_OTL_MovObjSelc/LM_OTL_MovObjInterestedSelc/LM_OTL_ObjSelcIndexCheck/HostObj1Check ==
  LM_OTL_MovObjValid : Inport
  Object_DX : Inport  Port=2
  HostObj1CheckInfo : Inport  Port=3
  If : If  IfExpression=u1 == 0
  If Action Subsystem : Subsystem  TreatAsAtomicUnit=on
  If Action Subsystem1 : Subsystem  TreatAsAtomicUnit=on
  Merge : Merge
  LM_OTLHostObj1Index : Outport
  wires:
  If Action Subsystem/1(LM_OTLHostObj1Index) -> Merge/1
  HostObj1CheckInfo/1 -> If/1, If Action Subsystem1/1(HostObj1CheckInfo)
  LM_OTL_MovObjValid/1 -> If Action Subsystem1/2(LM_OTL_MovObjValid)
  Merge/1 -> LM_OTLHostObj1Index/1
  If/1 -> If Action Subsystem/Action
  If/2 -> If Action Subsystem1/Action
  If Action Subsystem1/1(LM_OTLHostObj1Index) -> Merge/2
  Object_DX/1 -> If Action Subsystem1/3(Object_DX)

== system PubIfDecisionLM_MDL/Subsystem2/LM_OTL/LM_OTL_MovObjTrajRecord3/LM_OTL_MovObjSelc/LM_OTL_MovObjInterestedSelc/LM_OTL_ObjSelcIndexCheck/HostObj2Check ==
  LM_OTL_MovObjValid : Inport
  Object_DX : Inport  Port=2
  HostObj2CheckInfo : Inport  Port=3
  If : If  IfExpression=u1 == 0
  If Action Subsystem : Subsystem  TreatAsAtomicUnit=on
  If Action Subsystem1 : Subsystem  TreatAsAtomicUnit=on
  Merge : Merge
  LM_OTLHostObj2Index : Outport
  wires:
  If Action Subsystem/1(LM_OTLHostObj2Index) -> Merge/1
  HostObj2CheckInfo/1 -> If/1, If Action Subsystem1/1(LeObj1CheckInfo)
  LM_OTL_MovObjValid/1 -> If Action Subsystem1/2(LM_OTL_MovObjValid)
  Merge/1 -> LM_OTLHostObj2Index/1
  If/1 -> If Action Subsystem/Action
  If/2 -> If Action Subsystem1/Action
  If Action Subsystem1/1(LM_OTLLeObj1Index) -> Merge/2
  Object_DX/1 -> If Action Subsystem1/3(Object_DX)

== system PubIfDecisionLM_MDL/Subsystem2/LM_OTL/LM_OTL_MovObjTrajRecord3/LM_OTL_MovObjSelc/LM_OTL_MovObjInterestedSelc/LM_OTL_ObjSelcIndexCheck/LeObj1Check ==
  LM_OTL_MovObjValid : Inport
  Object_DX : Inport  Port=2
  LeObj1CheckInfo : Inport  Port=3
  If : If  IfExpression=u1 == 0
  If Action Subsystem : Subsystem  TreatAsAtomicUnit=on
  If Action Subsystem1 : Subsystem  TreatAsAtomicUnit=on
  Merge : Merge
  LM_OTLLeObj1Index : Outport
  wires:
  If Action Subsystem/1(LM_OTLLeObj1Index) -> Merge/1
  If/1 -> If Action Subsystem/Action
  If Action Subsystem1/1(LM_OTLLeObj1Index) -> Merge/2
  If/2 -> If Action Subsystem1/Action
  LM_OTL_MovObjValid/1 -> If Action Subsystem1/2(LM_OTL_MovObjValid)
  Merge/1 -> LM_OTLLeObj1Index/1
  LeObj1CheckInfo/1 -> If/1, If Action Subsystem1/1(LeObj1CheckInfo)
  Object_DX/1 -> If Action Subsystem1/3(Object_DX)

== system PubIfDecisionLM_MDL/Subsystem2/LM_OTL/LM_OTL_MovObjTrajRecord3/LM_OTL_MovObjSelc/LM_OTL_MovObjInterestedSelc/LM_OTL_ObjSelcIndexCheck/LeObj2Check ==
  LM_OTL_MovObjValid : Inport
  Object_DX : Inport  Port=2
  LeObj2CheckInfo : Inport  Port=3
  If : If  IfExpression=u1 == 0
  If Action Subsystem : Subsystem  TreatAsAtomicUnit=on
  If Action Subsystem1 : Subsystem  TreatAsAtomicUnit=on
  Merge : Merge
  LM_OTLLeObj2Index : Outport
  wires:
  If Action Subsystem/1(LM_OTLLeObj2Index) -> Merge/1
  LM_OTL_MovObjValid/1 -> If Action Subsystem1/2(LM_OTL_MovObjValid)
  If Action Subsystem1/1(LM_OTLLeObj2Index) -> Merge/2
  Object_DX/1 -> If Action Subsystem1/3(Object_DX)
  LeObj2CheckInfo/1 -> If/1, If Action Subsystem1/1(LeObj1CheckInfo)
  If/2 -> If Action Subsystem1/Action
  If/1 -> If Action Subsystem/Action
  Merge/1 -> LM_OTLLeObj2Index/1

== system PubIfDecisionLM_MDL/Subsystem2/LM_OTL/LM_OTL_MovObjTrajRecord3/LM_OTL_MovObjSelc/LM_OTL_MovObjInterestedSelc/LM_OTL_ObjSelcIndexCheck/RigObj1Check ==
  LM_OTL_MovObjValid : Inport
  Object_DX : Inport  Port=2
  RigObj1CheckInfo : Inport  Port=3
  If : If  IfExpression=u1 == 0
  If Action Subsystem : Subsystem  TreatAsAtomicUnit=on
  If Action Subsystem1 : Subsystem  TreatAsAtomicUnit=on
  Merge : Merge
  LM_OTLRigObj1Index : Outport
  wires:
  If Action Subsystem/1(LM_OTLLeObj1Index) -> Merge/1
  RigObj1CheckInfo/1 -> If/1, If Action Subsystem1/1(RigObj1CheckInfo)
  LM_OTL_MovObjValid/1 -> If Action Subsystem1/2(LM_OTL_MovObjValid)
  Merge/1 -> LM_OTLRigObj1Index/1
  If/1 -> If Action Subsystem/Action
  If/2 -> If Action Subsystem1/Action
  If Action Subsystem1/1(LM_OTLRigObj1Index) -> Merge/2
  Object_DX/1 -> If Action Subsystem1/3(Object_DX)

== system PubIfDecisionLM_MDL/Subsystem2/LM_OTL/LM_OTL_MovObjTrajRecord3/LM_OTL_MovObjSelc/LM_OTL_MovObjInterestedSelc/LM_OTL_ObjSelcIndexCheck/RigObj2Check ==
  LM_OTL_MovObjValid : Inport
  Object_DX : Inport  Port=2
  RigObj2CheckInfo : Inport  Port=3
  If : If  IfExpression=u1 == 0
  If Action Subsystem : Subsystem  TreatAsAtomicUnit=on
  If Action Subsystem1 : Subsystem  TreatAsAtomicUnit=on
  Merge : Merge
  LM_OTLRigObj2Index : Outport
  wires:
  If Action Subsystem/1(LM_OTLLeObj1Index) -> Merge/1
  RigObj2CheckInfo/1 -> If/1, If Action Subsystem1/1(RigObj2CheckInfo)
  LM_OTL_MovObjValid/1 -> If Action Subsystem1/2(LM_OTL_MovObjValid)
  Merge/1 -> LM_OTLRigObj2Index/1
  If/1 -> If Action Subsystem/Action
  If/2 -> If Action Subsystem1/Action
  If Action Subsystem1/1(LM_OTLRigObj2Index) -> Merge/2
  Object_DX/1 -> If Action Subsystem1/3(Object_DX)

== system PubIfDecisionLM_MDL/Subsystem2/LM_OTL/LM_OTL_MovObjTrajRecord3/LM_OTL_MovObjSelc/Subsystem3/LM_OTL_MovObjSelect/LM_OTL_ExistProbAssess ==
  Object_Fus_Type : Inport
  Object_ExistProb : Inport  Port=2
  If : If  IfExpression=u1==2|u1==4|u1==8  ElseIfExpressions=(u1==6|u1==10|u1==12|u1==14),(u1==3|u1==5|u1==7|u1==9|u1==11|u1==13|u1==15)
  Merge : Merge  Inputs=4
  MultiRader : Subsystem  TreatAsAtomicUnit=on
  Rader&Video : Subsystem  TreatAsAtomicUnit=on
  Rader&Video1 : Subsystem  TreatAsAtomicUnit=on
  Relational Operator : RelationalOperator  Operator=>  OutDataTypeStr=boolean  RndMeth=Simplest
  SingleRader : Subsystem  TreatAsAtomicUnit=on
  LM_OTL_ExistProbValid : Outport
  wires:
  Relational Operator/1 -> LM_OTL_ExistProbValid/1  "LM_OTL_ExistProbValid"
  Merge/1 -> Relational Operator/2
  Object_Fus_Type/1 -> If/1
  Object_ExistProb/1 -> Relational Operator/1
  If/1 -> SingleRader/Action
  If/2 -> MultiRader/Action
  If/3 -> Rader&Video/Action
  SingleRader/1(Out1) -> Merge/1
  MultiRader/1(Out1) -> Merge/2
  Rader&Video/1(Out1) -> Merge/3
  Rader&Video1/1(Out1) -> Merge/4
  If/4 -> Rader&Video1/Action

== system PubIfDecisionLM_MDL/Subsystem2/LM_OTL/LM_OTL_MovObjTrajRecord3/LM_OTL_MovObjSelc/Subsystem3/LM_OTL_MovObjSelect/LM_OTL_FusTypeAssess ==
  Object_Fus_Type : Inport
  Constant : Constant  Value=OFM_OBJ_FUSIONTYPE_E.INVALID
  Constant1 : Constant  Value=OFM_OBJ_FUSIONTYPE_E.FC
  Data Type Conversion : DataTypeConversion  OutDataTypeStr=Enum: OFM_OBJ_FUSIONTYPE_E
  Logical Operator : Logic  AllPortsSameDT=off  OutDataTypeStr=boolean
  Relational Operator : RelationalOperator  Operator=~=  OutDataTypeStr=boolean  RndMeth=Simplest
  Relational Operator1 : RelationalOperator  Operator=~=  OutDataTypeStr=boolean  RndMeth=Simplest
  LM_OTL_FusTypeValid : Outport
  wires:
  Constant1/1 -> Relational Operator1/2
  Constant/1 -> Relational Operator/2
  Data Type Conversion/1 -> Relational Operator/1, Relational Operator1/1
  Logical Operator/1 -> LM_OTL_FusTypeValid/1  "LM_OTL_FusTypeValid"
  Relational Operator1/1 -> Logical Operator/2
  Relational Operator/1 -> Logical Operator/1
  Object_Fus_Type/1 -> Data Type Conversion/1

== system PubIfDecisionLM_MDL/Subsystem2/LM_OTL/LM_OTL_MovObjTrajRecord3/LM_OTL_MovObjSelc/Subsystem3/LM_OTL_MovObjSelect/LM_OTL_MovDirAssess ==
  Object_Orientation : Inport
  Compare To Constant1 : simulink/Logic and Bit Operations/Compare To Constant  relop===  const=OFM_OBJ_ORIENTATION_E.NORTH  OutDataTypeStr=boolean
  Data Type Conversion : DataTypeConversion  OutDataTypeStr=Enum: OFM_OBJ_ORIENTATION_E
  LM_OTL_MovDirValid : Outport
  wires:
  Data Type Conversion/1 -> Compare To Constant1/1
  Compare To Constant1/1 -> LM_OTL_MovDirValid/1  "LM_OTL_MovDirValid"
  Object_Orientation/1 -> Data Type Conversion/1

== system PubIfDecisionLM_MDL/Subsystem2/LM_OTL/LM_OTL_MovObjTrajRecord3/LM_OTL_MovObjSelc/Subsystem3/LM_OTL_MovObjSelect/LM_OTL_MovStsAssess ==
  Object_MovingState : Inport
  Object_VX : Inport  Port=2
  vxvRefMs : Inport  Port=3
  Add : Sum
  Compare To Constant2 : simulink/Logic and Bit Operations/Compare To Constant  relop=>  const=P_LM_OTLObjSelectVxThre  OutDataTypeStr=boolean
  Constant : Constant  Value=OFM_OBJ_MOVINGSTATE_E.MOVING
  Constant1 : Constant  Value=OFM_OBJ_MOVINGSTATE_E.MOVING_SLOWLY
  Data Type Conversion : DataTypeConversion  OutDataTypeStr=Enum: OFM_OBJ_MOVINGSTATE_E
  Gain : Gain  Gain=3.6
  Logical Operator : Logic  AllPortsSameDT=off  OutDataTypeStr=boolean
  Logical Operator1 : Logic  Operator=OR  AllPortsSameDT=off  OutDataTypeStr=boolean
  Relational Operator : RelationalOperator  Operator===  OutDataTypeStr=boolean  RndMeth=Simplest
  Relational Operator1 : RelationalOperator  Operator===  OutDataTypeStr=boolean  RndMeth=Simplest
  LM_OTL_MovStsValid : Outport
  wires:
  Relational Operator1/1 -> Logical Operator1/2
  Relational Operator/1 -> Logical Operator1/1
  Constant1/1 -> Relational Operator1/2
  Constant/1 -> Relational Operator/2
  Data Type Conversion/1 -> Relational Operator/1, Relational Operator1/1
  Logical Operator/1 -> LM_OTL_MovStsValid/1  "LM_OTL_MovStsValid"
  Compare To Constant2/1 -> Logical Operator/2
  Gain/1 -> Compare To Constant2/1
  Add/1 -> Gain/1
  Logical Operator1/1 -> Logical Operator/1
  Object_MovingState/1 -> Data Type Conversion/1
  Object_VX/1 -> Add/1
  vxvRefMs/1 -> Add/2

== system PubIfDecisionLM_MDL/Subsystem2/LM_OTL/LM_OTL_MovObjTrajRecord3/LM_OTL_MovObjSelc/Subsystem3/LM_OTL_MovObjSelect/LM_OTL_ObjAgeAssess ==
  Object_Age : Inport
  Compare To Constant : simulink/Logic and Bit Operations/Compare To Constant  relop=>  const=P_LM_OTLObjSelectAgeThre  OutDataTypeStr=boolean
  LM_OTL_ObjAgeValid : Outport
  wires:
  Compare To Constant/1 -> LM_OTL_ObjAgeValid/1  "LM_OTL_ObjAgeValid"
  Object_Age/1 -> Compare To Constant/1

== system PubIfDecisionLM_MDL/Subsystem2/LM_OTL/LM_OTL_MovObjTrajRecord3/LM_OTL_MovObjSelc/Subsystem3/LM_OTL_MovObjSelect/LM_OTL_ObjDxAssess ==
  Object_DX : Inport
  vxvRefMs : Inport  Port=2
  1-D Lookup Table : Lookup_n-D  NumberOfTableDimensions=1  BreakpointsForDimension1=P_LM_OTLObjSelectDxAssessVx  Table=P_LM_OTLObjSelectDxThre  InternalRulePriority=Speed  RndMeth=Simplest  InputSameDT=on
  Logical Operator : Logic  Operator=NOT  AllPortsSameDT=off  OutDataTypeStr=boolean
  Relational Operator2 : RelationalOperator  Operator=>  OutDataTypeStr=boolean  RndMeth=Simplest
  LM_OTL_ObjDxValid : Outport
  wires:
  Relational Operator2/1 -> Logical Operator/1
  1-D Lookup Table/1 -> Relational Operator2/2
  Object_DX/1 -> Relational Operator2/1
  vxvRefMs/1 -> 1-D Lookup Table/1
  Logical Operator/1 -> LM_OTL_ObjDxValid/1  "LM_OTL_ObjDxValid"

== system PubIfDecisionLM_MDL/Subsystem2/LM_OTL/LM_OTL_MovObjTrajRecord3/LM_OTL_MovObjSelc/Subsystem3/LM_OTL_MovObjSelect/LM_OTL_ObjTypeAssess ==
  Object_Type : Inport
  Constant : Constant  Value=OFM_OBJ_TYPE_E.CAR  OutDataTypeStr=Enum: OFM_OBJ_TYPE_E
  Constant1 : Constant  Value=OFM_OBJ_TYPE_E.TRUCK  OutDataTypeStr=Enum: OFM_OBJ_TYPE_E
  Data Type Conversion : DataTypeConversion  OutDataTypeStr=Enum: OFM_OBJ_TYPE_E
  Logical Operator : Logic  Operator=OR  AllPortsSameDT=off  OutDataTypeStr=boolean
  Relational Operator : RelationalOperator  Operator===  OutDataTypeStr=boolean  RndMeth=Simplest
  Relational Operator1 : RelationalOperator  Operator===  OutDataTypeStr=boolean  RndMeth=Simplest
  LM_OTL_ObjTypeAssess : Outport
  wires:
  Data Type Conversion/1 -> Relational Operator/1, Relational Operator1/1
  Logical Operator/1 -> LM_OTL_ObjTypeAssess/1  "LM_OTL_ObjType"
  Constant/1 -> Relational Operator/2
  Constant1/1 -> Relational Operator1/2
  Relational Operator/1 -> Logical Operator/1
  Relational Operator1/1 -> Logical Operator/2
  Object_Type/1 -> Data Type Conversion/1

== system PubIfDecisionLM_MDL/Subsystem2/LM_OTL/LM_OTL_MovObjTrajRecord3/LM_OTL_MovObjSelc/Subsystem3/LM_OTL_MovObjSelect/LM_OTL_ObjVyAssess ==
  Object_VY : Inport
  Object_DX : Inport  Port=2
  1-D Lookup Table : Lookup_n-D  NumberOfTableDimensions=1  BreakpointsForDimension1=P_LM_OTLObjSelectVyAssessDx  Table=P_LM_OTLObjSelectVyThre  InternalRulePriority=Speed  RndMeth=Simplest  InputSameDT=on
  Abs : Abs
  Gain : Gain  Gain=3.6
  Relational Operator : RelationalOperator  Operator=<  OutDataTypeStr=boolean  RndMeth=Simplest
  LM_OTL_ObjVyValid : Outport
  wires:
  Abs/1 -> Gain/1
  Relational Operator/1 -> LM_OTL_ObjVyValid/1  "LM_OTL_ObjVyValid"
  1-D Lookup Table/1 -> Relational Operator/2
  Gain/1 -> Relational Operator/1
  Object_DX/1 -> 1-D Lookup Table/1
  Object_VY/1 -> Abs/1

== system PubIfDecisionLM_MDL/Subsystem2/LM_OTL/LM_OTL_MovObjTrajRecord3/LM_OTL_ObjStoreInfoCalc/LM_OTL_BufLe1InfoUpdate1/LM_OTL_BufLe1InfoUpdate/If Action Subsystem ==
  LM_OTLBufL1Objdx : Inport
  LM_OTLBufL1Objdy : Inport  Port=2
  LM_OTLBufL1EPPos : Inport  Port=3
  LM_OTLBufL1DxVectK1Adju : Inport  Port=4
  LM_OTLBufL1DyVectK1Adju : Inport  Port=5
  Action Port : ActionPort
  Assignment : Assignment  DiagnosticForDimensions=Warning  IndexOptions=Index vector (port)  Indices=1  OutputSizes=1
  Assignment1 : Assignment  DiagnosticForDimensions=Warning  IndexOptions=Index vector (port)  Indices=1  OutputSizes=1
  LM_OTLBufL1DxVect : Outport
  LM_OTLBufL1DyVect : Outport  Port=2
  wires:
  Assignment1/1 -> LM_OTLBufL1DyVect/1  "LM_OTLBufL1DyVect"
  Assignment/1 -> LM_OTLBufL1DxVect/1  "LM_OTLBufL1DxVect"
  LM_OTLBufL1Objdy/1 -> Assignment1/2
  LM_OTLBufL1DyVectK1Adju/1 -> Assignment1/1
  LM_OTLBufL1EPPos/1 -> Assignment/3, Assignment1/3
  LM_OTLBufL1Objdx/1 -> Assignment/2
  LM_OTLBufL1DxVectK1Adju/1 -> Assignment/1

== system PubIfDecisionLM_MDL/Subsystem2/LM_OTL/LM_OTL_MovObjTrajRecord3/LM_OTL_ObjStoreInfoCalc/LM_OTL_BufLe1InfoUpdate1/LM_OTL_BufLe1InfoUpdate/If Action Subsystem1 ==
  LM_OTLBufL1DxVectK1Adju : Inport
  LM_OTLBufL1DyVectK1Adju : Inport  Port=2
  Action Port : ActionPort
  Signal Conversion : SignalConversion  OverrideOpt=off
  Signal Conversion1 : SignalConversion  OverrideOpt=off
  LM_OTLBufL1DxVect : Outport
  LM_OTLBufL1DyVect : Outport  Port=2
  wires:
  Signal Conversion1/1 -> LM_OTLBufL1DyVect/1  "LM_OTLBufL1DyVect"
  Signal Conversion/1 -> LM_OTLBufL1DxVect/1  "LM_OTLBufL1DxVect"
  LM_OTLBufL1DyVectK1Adju/1 -> Signal Conversion1/1
  LM_OTLBufL1DxVectK1Adju/1 -> Signal Conversion/1

== system PubIfDecisionLM_MDL/Subsystem2/LM_OTL/LM_OTL_MovObjTrajRecord3/LM_OTL_ObjStoreInfoCalc/LM_OTL_BufLe1InfoUpdate1/LM_OTL_BufLe1StoreInfoCalc/LM_OTL_ObjSICCurLeObj1InBufLe1 ==
  LM_OTLCurLeLaObj1RcdFlg : Inport
  LM_OTLCurLeLaObj1ID : Inport  Port=2
  LM_OTLCurLeLaObj1Dx : Inport  Port=3
  LM_OTLCurLeLaObj1Dy : Inport  Port=4
  LM_OTLBufL1PNumK1 : Inport  Port=5
  LM_OTLBufL1SPPosK1 : Inport  Port=6
  LM_OTLBufL1EPPosK1 : Inport  Port=7
  Action Port : ActionPort
  LM_OTL_BufL1DxInfo : Subsystem
  LM_OTL_BufL1DyInfo : Subsystem
  LM_OTL_BufL1EPInfo : Subsystem
  LM_OTL_BufL1IDInfo : Subsystem
  LM_OTL_BufL1PNumInfo : Subsystem
  LM_OTL_BufL1SPInfo : Subsystem
  LM_OTL_BufL1UpdateFlg : Subsystem
  LM_OTLBufL1UpdateFlg : Outport
  LM_OTLBufL1ObjID : Outport  Port=2
  LM_OTLBufL1Objdx : Outport  Port=3
  LM_OTLBufL1Objdy : Outport  Port=4
  LM_OTLBufL1ObjTPNum : Outport  Port=5
  LM_OTLBufL1ObjTPSP : Outport  Port=6
  LM_OTLBufL1ObjTPEP : Outport  Port=7
  wires:
  LM_OTL_BufL1EPInfo/1(LM_OTLBufL1EPPos) -> LM_OTLBufL1ObjTPEP/1, [LM_OTLBufL1EPPos]
  [LM_OTLBufL1EPPos] -> LM_OTL_BufL1SPInfo/2(LM_OTLBufL1EPPos)
  LM_OTL_BufL1IDInfo/1(LM_OTLBufL1ObjID) -> LM_OTLBufL1ObjID/1
  LM_OTL_BufL1DxInfo/1(LM_OTLBufL1Objdx) -> LM_OTLBufL1Objdx/1
  LM_OTL_BufL1DyInfo/1(LM_OTLBufL1ObjDy) -> LM_OTLBufL1Objdy/1
  LM_OTL_BufL1PNumInfo/1(LM_OTLBufL1PNum) -> LM_OTLBufL1ObjTPNum/1
  LM_OTL_BufL1SPInfo/1(LM_OTLBufL1SPPos) -> LM_OTLBufL1ObjTPSP/1
  LM_OTL_BufL1UpdateFlg/1(LM_OTLBufL1UpdateFlg) -> LM_OTLBufL1UpdateFlg/1
  LM_OTLCurLeLaObj1RcdFlg/1 -> LM_OTL_BufL1EPInfo/1(LM_OTLCurLeLaObj1RcdFlg), LM_OTL_BufL1PNumInfo/2(LM_OTLCurLeLaObj1RcdFlg), LM_OTL_BufL1DyInfo/2(LM_OTLCurLeLaObj1RcdFlg), LM_OTL_BufL1DxInfo/2(LM_OTLCurLeLaObj1RcdFlg), LM_OTL_BufL1UpdateFlg/1(LM_OTLCurLeLaObj1RcdFlg)
  LM_OTLCurLeLaObj1ID/1 -> LM_OTL_BufL1IDInfo/1(LM_OTLCurLeLaObj1ID)
  LM_OTLCurLeLaObj1Dx/1 -> LM_OTL_BufL1DxInfo/1(LM_OTLCurLeLaObj1Dx)
  LM_OTLCurLeLaObj1Dy/1 -> LM_OTL_BufL1DyInfo/1(LM_OTLCurLeLaObj1Dy)
  LM_OTLBufL1PNumK1/1 -> LM_OTL_BufL1PNumInfo/1(LM_OTLBufL1PNumK1)
  LM_OTLBufL1SPPosK1/1 -> LM_OTL_BufL1SPInfo/1(LM_OTLBufL1SPPosK1)
  LM_OTLBufL1EPPosK1/1 -> LM_OTL_BufL1EPInfo/2(LM_OTLBufL1EPPosK1)

== system PubIfDecisionLM_MDL/Subsystem2/LM_OTL/LM_OTL_MovObjTrajRecord3/LM_OTL_ObjStoreInfoCalc/LM_OTL_BufLe1InfoUpdate1/LM_OTL_BufLe1StoreInfoCalc/LM_OTL_ObjSICCurLeObj2InBufLe1 ==
  LM_OTLCurLeLaObj2RcdFlg : Inport
  LM_OTLCurLeLaObj2ID : Inport  Port=2
  LM_OTLCurLeLaObj2Dx : Inport  Port=3
  LM_OTLCurLeLaObj2Dy : Inport  Port=4
  LM_OTLBufL1PNumK1 : Inport  Port=5
  LM_OTLBufL1SPPosK1 : Inport  Port=6
  LM_OTLBufL1EPPosK1 : Inport  Port=7
  Action Port : ActionPort
  LM_OTL_BufL1DxInfo : Subsystem
  LM_OTL_BufL1DyInfo : Subsystem
  LM_OTL_BufL1EPInfo : Subsystem
  LM_OTL_BufL1IDInfo : Subsystem
  LM_OTL_BufL1PNumInfo : Subsystem
  LM_OTL_BufL1SPInfo : Subsystem
  LM_OTL_BufL1UpdateFlg : Subsystem
  LM_OTLBufL1UpdateFlg : Outport
  LM_OTLBufL1ObjID : Outport  Port=2
  LM_OTLBufL1Objdx : Outport  Port=3
  LM_OTLBufL1Objdy : Outport  Port=4
  LM_OTLBufL1ObjTPNum : Outport  Port=5
  LM_OTLBufL1ObjTPSP : Outport  Port=6
  LM_OTLBufL1ObjTPEP : Outport  Port=7
  wires:
  LM_OTLBufL1PNumK1/1 -> LM_OTL_BufL1PNumInfo/1(LM_OTLBufL1PNumK1)
  LM_OTLCurLeLaObj2Dx/1 -> LM_OTL_BufL1DxInfo/1(LM_OTLCurLeLaObj1Dx)
  LM_OTL_BufL1IDInfo/1(LM_OTLBufL1ObjID) -> LM_OTLBufL1ObjID/1
  [LM_OTLBufL1EPPos] -> LM_OTL_BufL1SPInfo/2(LM_OTLBufL1EPPos)
  LM_OTL_BufL1PNumInfo/1(LM_OTLBufL1PNum) -> LM_OTLBufL1ObjTPNum/1
  LM_OTLCurLeLaObj2Dy/1 -> LM_OTL_BufL1DyInfo/1(LM_OTLCurLeLaObj1Dy)
  LM_OTL_BufL1DxInfo/1(LM_OTLBufL1Objdx) -> LM_OTLBufL1Objdx/1
  LM_OTLCurLeLaObj2RcdFlg/1 -> LM_OTL_BufL1EPInfo/1(LM_OTLCurLeLaObj1RcdFlg), LM_OTL_BufL1PNumInfo/2(LM_OTLCurLeLaObj1RcdFlg), LM_OTL_BufL1DyInfo/2(LM_OTLCurLeLaObj1RcdFlg), LM_OTL_BufL1DxInfo/2(LM_OTLCurLeLaObj1RcdFlg), LM_OTL_BufL1UpdateFlg/1(LM_OTLCurLeLaObj1RcdFlg)
  LM_OTL_BufL1SPInfo/1(LM_OTLBufL1SPPos) -> LM_OTLBufL1ObjTPSP/1
  LM_OTLCurLeLaObj2ID/1 -> LM_OTL_BufL1IDInfo/1(LM_OTLCurLeLaObj1ID)
  LM_OTL_BufL1DyInfo/1(LM_OTLBufL1ObjDy) -> LM_OTLBufL1Objdy/1
  LM_OTL_BufL1EPInfo/1(LM_OTLBufL1EPPos) -> LM_OTLBufL1ObjTPEP/1, [LM_OTLBufL1EPPos]
  LM_OTLBufL1EPPosK1/1 -> LM_OTL_BufL1EPInfo/2(LM_OTLBufL1EPPosK1)
  LM_OTL_BufL1UpdateFlg/1(LM_OTLBufL1UpdateFlg) -> LM_OTLBufL1UpdateFlg/1
  LM_OTLBufL1SPPosK1/1 -> LM_OTL_BufL1SPInfo/1(LM_OTLBufL1SPPosK1)

== system PubIfDecisionLM_MDL/Subsystem2/LM_OTL/LM_OTL_MovObjTrajRecord3/LM_OTL_ObjStoreInfoCalc/LM_OTL_BufLe1InfoUpdate1/LM_OTL_BufLe1StoreInfoCalc/LM_OTL_ObjSICNoCurObjInBufLe1 ==
  LM_OTLCurLeLaObj1Index : Inport
  LM_OTLCurLeLaObj2Index : Inport  Port=2
  LM_OTLCurLeLaObj1RcdedFlg : Inport  Port=3
  LM_OTLCurLeLaObj1ID : Inport  Port=4
  LM_OTLCurLeLaObj2ID : Inport  Port=5
  LM_OTLCurLeLaObj1Dx : Inport  Port=6
  LM_OTLCurLeLaObj2Dx : Inport  Port=7
  LM_OTLCurLeLaObj1Dy : Inport  Port=8
  LM_OTLCurLeLaObj2Dy : Inport  Port=9
  LM_OTLBufL1LastTPValid : Inport  Port=10
  LM_OTLBufL1LastEPPos : Inport  Port=11
  Action Port : ActionPort
  LM_OTL_BufL1DxInfo : Subsystem
  LM_OTL_BufL1DyInfo : Subsystem
  LM_OTL_BufL1EPInfo : Subsystem
  LM_OTL_BufL1IDInfo : Subsystem
  LM_OTL_BufL1PNumInfo : Subsystem
  LM_OTL_BufL1SPInfo : Subsystem
  LM_OTLBufL1UpdateFlg : Outport
  LM_OTLBufL1ObjID : Outport  Port=2
  LM_OTLBufL1Objdx : Outport  Port=3
  LM_OTLBufL1Objdy : Outport  Port=4
  LM_OTLBufL1ObjTPNum : Outport  Port=5
  LM_OTLBufL1ObjTPSP : Outport  Port=6
  LM_OTLBufL1ObjTPEP : Outport  Port=7
  wires:
  LM_OTL_BufL1IDInfo/2(LM_OTLBufL1ObjID) -> LM_OTLBufL1ObjID/1
  LM_OTL_BufL1DxInfo/1(LM_OTLBufL1Objdx) -> LM_OTLBufL1Objdx/1
  LM_OTL_BufL1DyInfo/1(LM_OTLBufL1Objdy) -> LM_OTLBufL1Objdy/1
  LM_OTL_BufL1PNumInfo/1(LM_OTLBufL1TPNum) -> LM_OTLBufL1ObjTPNum/1
  LM_OTL_BufL1SPInfo/1(LM_OTLBufL1SPPos) -> LM_OTL_BufL1EPInfo/1(LM_OTLBufL1SPPos), LM_OTLBufL1ObjTPSP/1
  LM_OTL_BufL1EPInfo/1(LM_OTLBufL1EPPos) -> LM_OTLBufL1ObjTPEP/1
  LM_OTLCurLeLaObj1Index/1 -> LM_OTL_BufL1SPInfo/1(LM_OTLCurLeLaObj1Index), LM_OTL_BufL1PNumInfo/1(LM_OTLCurLeLaObj1Index), LM_OTL_BufL1DyInfo/1(LM_OTLCurLeLaObj1Index), LM_OTL_BufL1DxInfo/1(LM_OTLCurLeLaObj1Index), LM_OTL_BufL1IDInfo/1(LM_OTLCurLeLaObj1Index)
  LM_OTLCurLeLaObj1ID/1 -> LM_OTL_BufL1SPInfo/2(LM_OTLCurLeLaObj2Index), LM_OTL_BufL1PNumInfo/2(LM_OTLCurLeLaObj2Index), LM_OTL_BufL1DyInfo/2(LM_OTLCurLeLaObj2Index), LM_OTL_BufL1DxInfo/2(LM_OTLCurLeLaObj2Index), LM_OTL_BufL1IDInfo/2(LM_OTLCurLeLaObj2Index)
  LM_OTLCurLeLaObj1RcdedFlg/1 -> LM_OTL_BufL1SPInfo/3(LM_OTLCurLeLaObj1RcdedFlg), LM_OTL_BufL1PNumInfo/3(LM_OTLCurLeLaObj1RcdedFlg), LM_OTL_BufL1DyInfo/3(LM_OTLCurLeLaObj1RcdedFlg), LM_OTL_BufL1DxInfo/3(LM_OTLCurLeLaObj1RcdedFlg), LM_OTL_BufL1IDInfo/3(LM_OTLCurLeLaObj1RcdedFlg)
  LM_OTLCurLeLaObj2Index/1 -> LM_OTL_BufL1IDInfo/4(LM_OTLCurLeLaObj1ID)
  LM_OTLCurLeLaObj2ID/1 -> LM_OTL_BufL1IDInfo/5(LM_OTLCurLeLaObj2ID)
  LM_OTLCurLeLaObj1Dx/1 -> LM_OTL_BufL1DxInfo/4(LM_OTLCurLeLaObj1Dx)
  LM_OTLCurLeLaObj2Dx/1 -> LM_OTL_BufL1DxInfo/5(LM_OTLCurLeLaObj2Dx)
  LM_OTLCurLeLaObj2Dy/1 -> LM_OTL_BufL1DyInfo/5(LM_OTLCurLeLaObj2Dy)
  LM_OTLCurLeLaObj1Dy/1 -> LM_OTL_BufL1DyInfo/4(LM_OTLCurLeLaObj1Dy)
  LM_OTLBufL1LastTPValid/1 -> LM_OTL_BufL1SPInfo/4(LM_OTLBufL1LastTPValid)
  LM_OTLBufL1LastEPPos/1 -> LM_OTL_BufL1SPInfo/5(LM_OTLBufL1LastEPPos)
  LM_OTL_BufL1IDInfo/1(LM_OTLBufL1UpdateFlg) -> LM_OTLBufL1UpdateFlg/1

== system PubIfDecisionLM_MDL/Subsystem2/LM_OTL/LM_OTL_MovObjTrajRecord3/LM_OTL_ObjStoreInfoCalc/Subsystem/LM_OTL_BufLastTPInfo/LM_OTL_BufL1LastTPInfoAdju1 ==
  note: P_LM_OTLBufRearDisThre
  note: P_LM_OTLBufPNum
  note: P_LM_OTLBufTPMinNum
  LM_OTLBufL1EPPos : Inport
  LM_OTLBufL1DxVect : Inport  Port=2
  LM_OTLBufL1LastTPValid : Inport  Port=3
  LM_OTLBufL1LastPNum : Inport  Port=4
  LM_OTLBufL1LastSPPos : Inport  Port=5
  LM_OTLBufL1LastEPPos : Inport  Port=6
  Add : Sum
  Constant : Constant  Value=0  OutDataTypeStr=uint8
  Constant1 : Constant  OutDataTypeStr=uint8
  Constant2 : Constant  Value=80  OutDataTypeStr=uint8
  Constant3 : Constant  OutDataTypeStr=uint8
  Constant4 : Constant  OutDataTypeStr=uint8
  Constant5 : Constant  Value=15
  Constant6 : Constant  Value=-60  OutDataTypeStr=single
  Index Vector : MultiPortSwitch  Inputs=1
  Logical Operator1 : Logic  Operator=OR  AllPortsSameDT=off  OutDataTypeStr=boolean
  Logical Operator2 : Logic  Operator=OR  AllPortsSameDT=off  OutDataTypeStr=boolean
  Relational Operator1 : RelationalOperator  Operator===  OutDataTypeStr=boolean  RndMeth=Simplest
  Relational Operator2 : RelationalOperator  Operator=>  OutDataTypeStr=boolean  RndMeth=Simplest
  Relational Operator3 : RelationalOperator  Operator=<  OutDataTypeStr=boolean  RndMeth=Simplest
  Relational Operator4 : RelationalOperator  Operator=<=  OutDataTypeStr=boolean  RndMeth=Simplest
  Saturation : Saturate  UpperLimit=80  LowerLimit=0
  Subtract : Sum  Inputs=+-
  Switch{1..6} (6 alike) : Switch  Criteria=u2 ~= 0
  LM_OTLBufL1LastTPValidAdju : Outport
  LM_OTLBufL1LastPNumAdju : Outport  Port=2
  LM_OTLBufL1LastSPPosAdju : Outport  Port=3
  LM_OTLBufL1LastEPPosAdju : Outport  Port=4
  wires:
  Switch6/1 -> LM_OTLBufL1LastEPPosAdju/1
  LM_OTLBufL1LastEPPos/1 -> Switch6/3
  Switch4/1 -> LM_OTLBufL1LastSPPosAdju/1
  Switch5/1 -> LM_OTLBufL1LastPNumAdju/1
  Constant/1 -> Switch4/1, Switch5/1, Switch6/1
  Relational Operator4/1 -> Logical Operator2/2
  Relational Operator1/1 -> Logical Operator2/1
  Constant6/1 -> Relational Operator4/2
  Index Vector/1 -> Relational Operator4/1
  LM_OTLBufL1DxVect/1 -> Index Vector/2
  Logical Operator1/1 -> Switch4/2, Switch5/2, LM_OTLBufL1LastTPValidAdju/1, Switch6/2
  LM_OTLBufL1LastTPValid/1 -> Logical Operator1/2
  Relational Operator3/1 -> Logical Operator1/1
  Constant5/1 -> Relational Operator3/2
  Switch3/1 -> Relational Operator3/1, Switch5/3
  Saturation/1 -> Switch3/1
  Subtract/1 -> Saturation/1
  Constant4/1 -> Subtract/2
  LM_OTLBufL1LastPNum/1 -> Switch3/3, Subtract/1
  Switch2/1 -> Switch1/1
  Constant3/1 -> Switch2/1
  Switch1/1 -> Switch4/3
  Relational Operator2/1 -> Switch2/2
  Constant2/1 -> Relational Operator2/2
  Add/1 -> Switch2/3, Relational Operator2/1
  Constant1/1 -> Add/2
  Logical Operator2/1 -> Switch1/2, Switch3/2
  LM_OTLBufL1LastSPPos/1 -> Add/1, Relational Operator1/2, Index Vector/1, Switch1/3
  LM_OTLBufL1EPPos/1 -> Relational Operator1/1
